simulink model "I_ARX"  (R2015a)
settings: Solver=ode45  StartTime=0.0  StopTime=1000  RelTol=1e-3
values from neighbouring files (symbols this model uses):
  lambda = 0.99    [generar_prbs.m]
settings Model: Creator=n221  LastModifiedBy=ARTURO

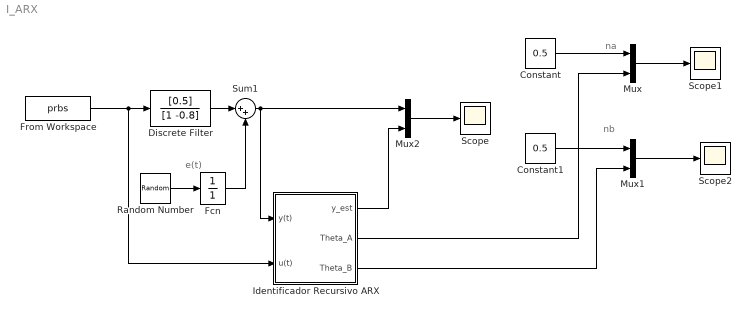
== system I_ARX ==
  note: nb
  note: na
  note: e(t)
  " Fcn" : DiscreteTransferFcn  Denominator=[1]
  Constant : Constant  Value=0.5
  Constant1 : Constant  Value=0.5
  Discrete Filter : DiscreteFilter  Numerator=[0.5]  Denominator=[1 -0.8]  SampleTime=0.01
  From Workspace : FromWorkspace  VariableName=prbs  SampleTime=0.01
  Identificador Recursivo ARX : Subsystem
  Mux : Mux  Inputs=2
  Mux1 : Mux  Inputs=2
  Mux2 : Mux  Inputs=2
  Random Number : RandomNumber  SampleTime=0.1
  Scope : Scope
  Scope1 : Scope
  Scope2 : Scope
      settings: TimeRange=10  SaveName=ScopeData2
  Sum1 : Sum  Inputs=|++
  wires:
  From Workspace/1 -> Discrete Filter/1, Identificador Recursivo ARX/2(u(t))
  Constant/1 -> Mux/1
  Constant1/1 -> Mux1/1
  Mux1/1 -> Scope2/1
  Mux/1 -> Scope1/1
  Identificador Recursivo ARX/2(Theta_A) -> Mux/2
  Identificador Recursivo ARX/3("Theta_B ") -> Mux1/2
  Identificador Recursivo ARX/1(y_est) -> Mux2/2
  Mux2/1 -> Scope/1
  Discrete Filter/1 -> Sum1/1
  Random Number/1 -> " Fcn"/1
  Sum1/1 -> Mux2/1, Identificador Recursivo ARX/1(y(t))
  " Fcn"/1 -> Sum1/2

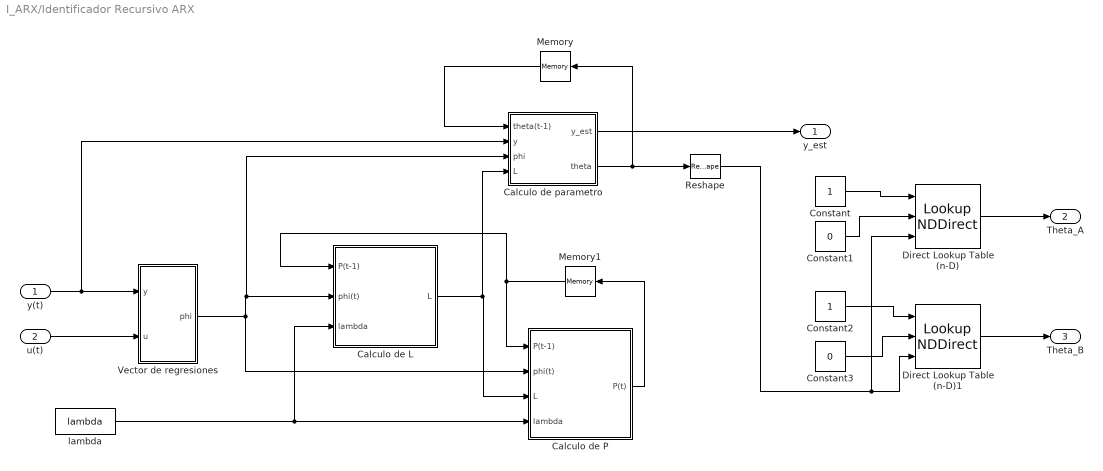
== system I_ARX/Identificador Recursivo ARX ==
  y(t) : Inport
  u(t) : Inport  Port=2
  Calculo de L : Subsystem
  Calculo de P : Subsystem
  Calculo de parametro : Subsystem
  Constant : Constant
  Constant1 : Constant  Value=0
  Constant2 : Constant
  Constant3 : Constant  Value=0
  Direct Lookup Table (n-D) : LookupNDDirect  TableIsInput=on  Table=[4 5 ;16 19 ]  DiagnosticForOutOfRangeInput=Error
  Direct Lookup Table (n-D)1 : LookupNDDirect  TableIsInput=on  Table=[4 5 ;16 19 ]  DiagnosticForOutOfRangeInput=Error
  Memory : Memory
  Memory1 : Memory  X0=1e6*eye(2)
  Reshape : Reshape  OutputDimensionality=Column vector (2-D)
  Vector de regresiones : Subsystem
  lambda : Constant  Value=lambda
  y_est : Outport
  Theta_A : Outport  Port=2
  "Theta_B " : Outport  Port=3
  wires:
  lambda/1 -> Calculo de P/4(lambda), Calculo de L/3(lambda)
  y(t)/1 -> Calculo de parametro/2(y), Vector de regresiones/1(y)
  u(t)/1 -> Vector de regresiones/2(u)
  Calculo de parametro/2(theta) -> Memory/1, Reshape/1
  Memory/1 -> Calculo de parametro/1(theta(t-1))
  Calculo de L/1(L) -> Calculo de parametro/4(L), Calculo de P/3(L)
  Calculo de P/1(P(t)) -> Memory1/1
  Memory1/1 -> Calculo de P/1(P(t-1)), Calculo de L/1(P(t-1))
  Vector de regresiones/1(phi) -> Calculo de parametro/3(phi), Calculo de L/2(phi(t)), Calculo de P/2(phi(t))
  Calculo de parametro/1(y_est) -> y_est/1
  Constant1/1 -> Direct Lookup Table (n-D)/2
  Constant/1 -> Direct Lookup Table (n-D)/1
  Constant2/1 -> Direct Lookup Table (n-D)1/1
  Constant3/1 -> Direct Lookup Table (n-D)1/2
  Reshape/1 -> Direct Lookup Table (n-D)/3, Direct Lookup Table (n-D)1/3
  Direct Lookup Table (n-D)/1 -> Theta_A/1
  Direct Lookup Table (n-D)1/1 -> "Theta_B "/1

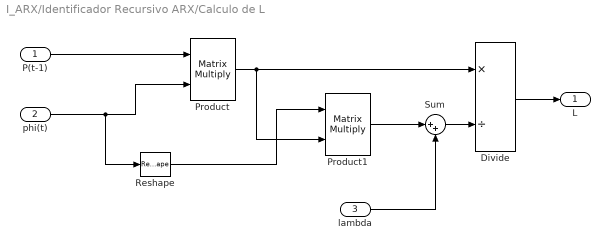
== system I_ARX/Identificador Recursivo ARX/Calculo de L ==
  P(t-1) : Inport
  phi(t) : Inport  Port=2
  lambda : Inport  Port=3
  Divide : Product  Inputs=*/
  Product : Product  Multiplication=Matrix(*)
  Product1 : Product  Multiplication=Matrix(*)
  Reshape : Reshape  OutputDimensionality=Row vector (2-D)
  Sum : Sum  Inputs=|++
  L : Outport
  wires:
  phi(t)/1 -> Reshape/1, Product/2
  Reshape/1 -> Product1/1
  Product/1 -> Product1/2, Divide/1
  Product1/1 -> Sum/1
  P(t-1)/1 -> Product/1
  lambda/1 -> Sum/2
  Sum/1 -> Divide/2
  Divide/1 -> L/1

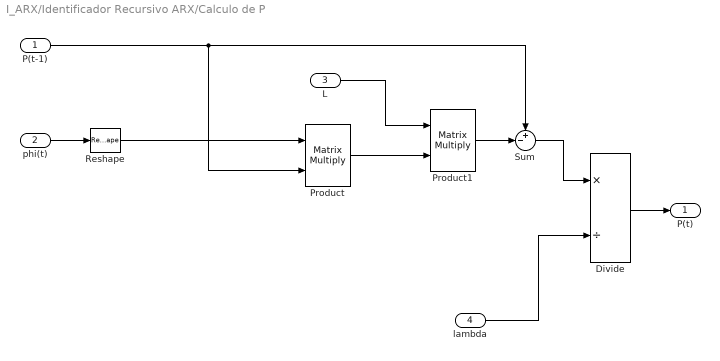
== system I_ARX/Identificador Recursivo ARX/Calculo de P ==
  P(t-1) : Inport
  phi(t) : Inport  Port=2
  L : Inport  Port=3
  lambda : Inport  Port=4
  Divide : Product  Inputs=*/
  Product : Product  Multiplication=Matrix(*)
  Product1 : Product  Multiplication=Matrix(*)
  Reshape : Reshape  OutputDimensionality=Row vector (2-D)
  Sum : Sum  Inputs=+-|
  P(t) : Outport
  wires:
  Reshape/1 -> Product/1
  Divide/1 -> P(t)/1
  lambda/1 -> Divide/2
  Product1/1 -> Sum/2
  P(t-1)/1 -> Product/2, Sum/1
  L/1 -> Product1/1
  Product/1 -> Product1/2
  phi(t)/1 -> Reshape/1
  Sum/1 -> Divide/1

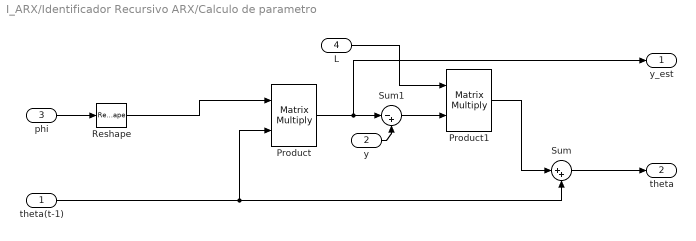
== system I_ARX/Identificador Recursivo ARX/Calculo de parametro ==
  theta(t-1) : Inport
  y : Inport  Port=2
  phi : Inport  Port=3
  L : Inport  Port=4
  Product : Product  Multiplication=Matrix(*)
  Product1 : Product  Multiplication=Matrix(*)
  Reshape : Reshape  OutputDimensionality=Row vector (2-D)
  Sum : Sum  Inputs=|++
  Sum1 : Sum  Inputs=|-+
  y_est : Outport
  theta : Outport  Port=2
  wires:
  phi/1 -> Reshape/1
  Reshape/1 -> Product/1
  theta(t-1)/1 -> Product/2, Sum/2
  L/1 -> Product1/1
  y/1 -> Sum1/2
  Product/1 -> y_est/1, Sum1/1
  Sum/1 -> theta/1
  Sum1/1 -> Product1/2
  Product1/1 -> Sum/1

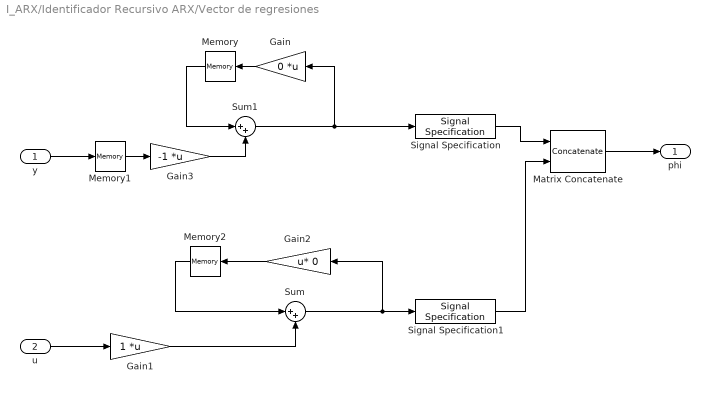
== system I_ARX/Identificador Recursivo ARX/Vector de regresiones ==
  y : Inport
  u : Inport  Port=2
  Gain : Gain  Gain=0  Multiplication=Matrix(K*u)
  Gain1 : Gain  Multiplication=Matrix(K*u)
  Gain2 : Gain  Gain=0  Multiplication=Matrix(u*K)
  Gain3 : Gain  Gain=-1  Multiplication=Matrix(K*u)
  Matrix Concatenate : Concatenate  Mode=Multidimensional array
  Memory : Memory
  Memory1 : Memory
  Memory2 : Memory
  Signal Specification : SignalSpecification  Dimensions=[1 1]
  Signal Specification1 : SignalSpecification  Dimensions=[1 1]
  Sum : Sum  Inputs=|++
  Sum1 : Sum  Inputs=|++
  phi : Outport
  wires:
  Gain/1 -> Memory/1
  y/1 -> Memory1/1
  u/1 -> Gain1/1
  Gain1/1 -> Sum/2
  Gain2/1 -> Memory2/1
  Memory2/1 -> Sum/1
  Signal Specification1/1 -> Matrix Concatenate/2
  Signal Specification/1 -> Matrix Concatenate/1
  Matrix Concatenate/1 -> phi/1
  Memory1/1 -> Gain3/1
  Gain3/1 -> Sum1/2
  Sum1/1 -> Gain/1, Signal Specification/1
  Memory/1 -> Sum1/1
  Sum/1 -> Gain2/1, Signal Specification1/1
